simulink model "car_control_alert"  (R2023a)
settings: Solver=VariableStepAuto  StartTime=0.0  StopTime=10.0  RelTol=1e-3
undefined symbols (not defined in the file or in its folder): magnitude
libraries: simulink x1
settings Model: Creator=15113  LastModifiedBy=15113

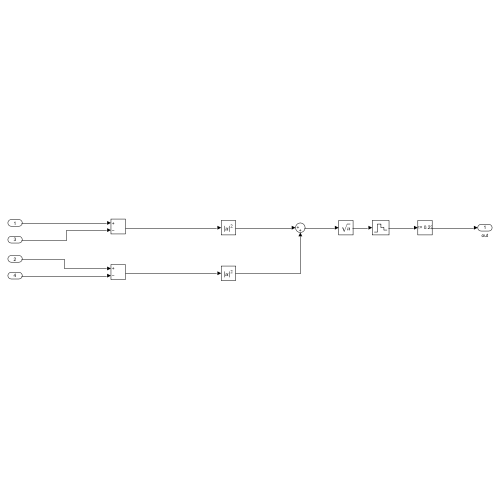
[thumbnail: Simulink's stored preview of the top-level diagram]
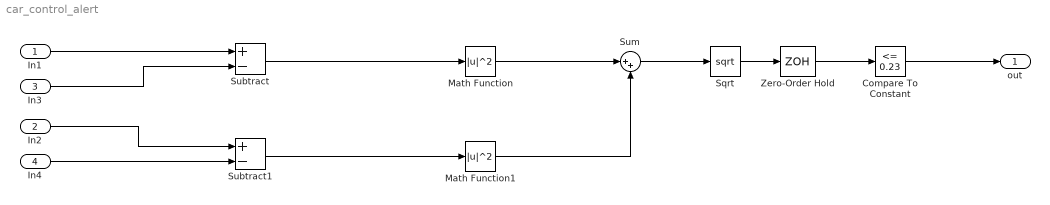
== system car_control_alert ==
  In1 : Inport
  In2 : Inport  Port=2
  In3 : Inport  Port=3
  In4 : Inport  Port=4
  Compare To Constant : simulink/Logic and Bit Operations/Compare To Constant  relop=<=  const=0.23  OutDataTypeStr=boolean
  Math Function : Math  Operator=magnitude^2
  Math Function1 : Math  Operator=magnitude^2
  Sqrt : Sqrt
  Subtract : Sum  Inputs=+-
  Subtract1 : Sum  Inputs=+-
  Sum : Sum  Inputs=|++
  Zero-Order Hold : ZeroOrderHold  SampleTime=0.25
  out : Outport
  wires:
  In1/1 -> Subtract/1
  In2/1 -> Subtract1/1
  In3/1 -> Subtract/2
  In4/1 -> Subtract1/2
  Subtract/1 -> Math Function/1
  Subtract1/1 -> Math Function1/1
  Math Function/1 -> Sum/1
  Math Function1/1 -> Sum/2
  Sum/1 -> Sqrt/1
  Sqrt/1 -> Zero-Order Hold/1
  Zero-Order Hold/1 -> Compare To Constant/1
  Compare To Constant/1 -> out/1
